simulink model "afe_abc_inv_psm"  (R2025b)
settings: Solver=ode1  StartTime=0.0  StopTime=simlength  FixedStep=tc  MaxStep=tc
values from neighbouring files (symbols this model uses):
  Adrso = eye(2) + Arso*ts_afe    [init_model.m]
  afe_pwm_phase_shift_mod1 = 0    [init_model.m]
  afe_pwm_phase_shift_mod2 = 0    [init_model.m]
  Aresd = eye(2) + Ares*ts_afe    [init_model.m]
  Bresd = Bres*ts_afe    [init_model.m]
  Cresd = Cres    [init_model.m]
  Crso = [1 0]    [init_model.m]
  CTRPIFF_CLIP_RELEASE = 0.001    [init_model.m]
  deepNEGeta = 0.5    [init_model.m]
  deepNEGxi = 0    [init_model.m]
  deepPOSxi = 0.5    [init_model.m]
  emf_fb_p = 0.2    [init_model.m]
  emf_fb_p_ccaller_1 = emf_fb_p    (= 0.2)    [init_model.m]
  emf_fb_p_ccaller_2 = emf_fb_p    (= 0.2)    [init_model.m]
  emf_p = emf_fb_p*4/10    (= 0.08)    [init_model.m]
  emf_p_ccaller_1 = emf_fb_p_ccaller_1*4/10    (= 0.08)    [init_model.m]
  emf_p_ccaller_2 = emf_fb_p_ccaller_2*4/10    (= 0.08)    [init_model.m]
  g0_161Hz = fcut_161Hz_flt * ts_afe * 2*pi    (= 0.126449104307)    [init_model.m]
  g0_1Hz = fcut_1Hz_flt * ts_afe * 2*pi    (= 0.000785398163397)    [init_model.m]
  g0_500Hz = fcut_500Hz_flt * ts_afe * 2*pi    (= 0.392699081699)    [init_model.m]
  g1_161Hz = 1 - g0_161Hz    (= 0.873550895693)    [init_model.m]
  g1_1Hz = 1 - g0_1Hz    (= 0.999214601837)    [init_model.m]
  g1_500Hz = 1 - g0_500Hz    (= 0.607300918301)    [init_model.m]
  i_grid_neg_eta_lim = 0.5    [init_model.m]
  i_grid_neg_eta_red_lim = 0.1    [init_model.m]
  i_grid_neg_xi_lim = 0.5    [init_model.m]
  i_grid_neg_xi_red_lim = 0.1    [init_model.m]
  i_grid_pos_eta_lim = 1    [init_model.m]
  i_grid_pos_eta_red_lim = 0.1    [init_model.m]
  id_lim = 0.35    [init_model.m]
  ieta_neg_ref_lim = 0.5    [init_model.m]
  ieta_pos_ref_lim = 1.0    (= 1)    [init_model.m]
  Igrid_phase_normalization_factor = 250e3/Vphase2/3/0.9*sqrt(2)    [init_model.m]
  inv_pwm_phase_shift_mod1 = 0    [init_model.m]
  iq_lim = 1.4    [init_model.m]
  ixi_pos_ref_lim = 1.6    [init_model.m]
  k_frt_ref = 2    [init_model.m]
  kg = Kobs(1)    [init_model.m]
  ki_afe = 45    [init_model.m]
  ki_align = 0.1    [init_model.m]
  ki_i = 18    [init_model.m]
  ki_rc_neg_grid = ki_rc_grid    (= 35)    [init_model.m]
  ki_rc_pos_grid = ki_rc_grid    (= 35)    [init_model.m]
  ki_vs = 35    [init_model.m]
  ki_w = 18    [init_model.m]
  kp_afe = 0.6    [init_model.m]
  kp_align = 0.6    [init_model.m]
  kp_i = 0.25    [init_model.m]
  kp_rc_neg_grid = kp_rc_grid    (= 0.35)    [init_model.m]
  kp_rc_pos_grid = kp_rc_grid    (= 0.35)    [init_model.m]
  kp_vs = 0.85    [init_model.m]
  kp_w = 2.5    [init_model.m]
  kw = Kobs(2)    [init_model.m]
  l1 = Kd(2)    [init_model.m]
  l2 = Kd(1)    [init_model.m]
  Ldrso = acker(Adrso',Crso',polesdrso)'    [init_model.m]
  lim_down_align = -0.2    [init_model.m]
  lim_up_align = 0.2    [init_model.m]
  mavarage_filter_frequency_base_order = 2    [init_model.m]
  motorc_m_scale = 2/3*Vdc_bez/ubez    [init_model.m]
  n1 = rms_perios/f_grid/ts_afe    [init_model.m]
  n10 = rms_perios/f_grid/ts_afe    [init_model.m]
  number_of_modules = 2    [init_model.m]
  omega_m_sim = omega_m_bez    [init_model.m]
  pll_i1 = 80    [init_model.m]
  pll_i1_ddsrt = pll_i1/2    (= 40)    [init_model.m]
  pll_p = 1    [init_model.m]
  pll_p_ddsrt = pll_p/2    (= 0.5)    [init_model.m]
  pll_p_frt = 0.2    [init_model.m]
  settle_time = 0.15    [init_model.m]
  simlength = 2    [init_model.m]
  start_time_LVRT = 2.0    (= 2)    [init_model.m]
  tc = ts_afe/200    (= 6.25e-07)    [init_model.m]
  time_aux_power_supply_fault = 1e3    (= 1000)    [init_model.m]
  time_gain_afe_module_1 = 1.0    (= 1)    [init_model.m]
  time_gain_afe_module_2 = 1.0    (= 1)    [init_model.m]
  time_gain_inv_module_1 = 1.0    (= 1)    [init_model.m]
  time_gain_inv_module_2 = 1.0    (= 1)    [init_model.m]
  time_phase_fault = 1e3    (= 1000)    [init_model.m]
  time_start_motor_control = 0.035    [init_model.m]
  transmission_delay = 125e-6*2    (= 0.00025)    [init_model.m]
  ts_afe = 1/fPWM_AFE/2    (= 0.000125)    [init_model.m]
  ts_inv = 1/fPWM_INV/2    (= 0.000125)    [init_model.m]
  Vdc_norm_ref = Vdc_ref/Vdc_nom    [init_model.m]
  Vdc_ref = 1070    [init_model.m]
  Vgrid_phase_normalization_factor = Vphase2*sqrt(2)    [init_model.m]
  w_grid = 2*pi*f_grid    [init_model.m]
undefined symbols (not defined in the file or in its folder): Amplitude_U, Amplitude_V, Amplitude_W, end_time_LVRT, ibez, La, Lb, Ld_norm, Lq_norm, Ls_norm, magnitude, omega_bez, omega_grid_emulator_nom, omega_grid_nom, omega_m_bez, Phase_shift, psi_bez, psi_m, psi_m_norm, rpm_base, rpm_bez, Rs, Rs_norm, t_ramp, tau_bez, torque_base, ubez, ugrid_factor, V_phase_normalization_factor, Vdc_bez, Vemu_ref_norm, vn_eta_pu, vn_xi_pu, vp_xi_pu
libraries: fl_lib x215, nesl_utility x107, simulink x22, cstblocks x20, threephase_inductor_lib x4, three_phase_pwm_modulator x4, single_phase_transformer_lib x3, power_meter_iec x1, flexshaft_lib x1, psm x1
(part 5 of 18)

== system afe_abc_inv_psm/afe_abc_inv_psm_mod2/inverter/inverter ==
  duties_uvw : Inport
  Bus Selector : BusSelector  OutputSignals=gate_cmd_Q1,gate_cmd_Q2,gate_cmd_Q3,gate_cmd_Q4,gate_cmd_Q5,gate_cmd_Q6
  Current Sensor1 : fl_lib/Electrical/Electrical Sensors/Current Sensor
  Product{,1..5} (6 alike) : Product
  Simulink-PS Converter{,1..5} (6 alike) : nesl_utility/Simulink-PS Converter  PhysicalDomain=network_engine_domain  SubClassName=ps_input  LeftPortType=input  RightPortType=output  PseudoPeriodic=off  Frequencies=[]  NoiseDistribution=none  NoiseParameters=[]  Unit=1  AffineConversion=on  FilteringAndDerivatives=provide  SimscapeFilterOrder=1  InputFilterTimeConstant=0.001  UdotUserProvided=0
  Step : Step  Time=time_aux_power_supply_fault  Before=1  After=0  SampleTime=0
  ileg_dc_inv : nesl_utility/PS-Simulink Converter  PhysicalDomain=network_engine_domain  SubClassName=ps_output  LeftPortType=input  RightPortType=output  PseudoPeriodic=off  Frequencies=[]  VectorFormat=1-D array  Unit=A  AffineConversion=on
  sv_pwm : Subsystem
  switch_1 : Subsystem
      settings: PortSchema="{\"entries\":[{\"content\":{\"sides\":[{\"content\":{\"connectorIds\":[\"LConn1\"]},\"type\":\"ConnectorPlacement.EquallySpacedRectSide\",\"uuid\":\"9277da8d-d460-43e6-8478-dd662f15d226\"},{\"content\":{\"connectorIds\":[],\"side\":\"RIGHT\"},\"type\":\"ConnectorPlacement.EquallySpacedRectSide\",\"uuid\":\"a7ece396-f1d9-4f4f-a05b-db1fc65d6e1d\"},{\"content\":{\"connectorIds\":[\"LConn2\"],\"side\":\"TOP\"},\"type\":\"ConnectorPlacement.EquallySpacedRectSide\",\"uuid\":\"fdd70777-e9cf-4317-afb6-cae87f75d5b0\"},{\"content\":{\"connectorIds\":[\"RConn1\"],\"side\":\"BOTTOM\"},\"type\":\"ConnectorPlacement.EquallySpacedRectSide\",\"uuid\":\"2353ed68-b1a1-4775-9ca9-31e268d5443b\"}]},\"type\":\"ConnectorPlacement.EquallySpacedConnector\",\"uuid\":\"d5479f4c-4e65-4791-adcb-73df11f88590\"}],\"packageUris\":[\"http://schema.mathworks.com/mf0/Connector/R2020b\"],\"version\":\"1.0\"}"
  switch_2 : Subsystem
      settings: PortSchema="{\"entries\":[{\"content\":{\"sides\":[{\"content\":{\"connectorIds\":[\"LConn1\"]},\"type\":\"ConnectorPlacement.EquallySpacedRectSide\",\"uuid\":\"9277da8d-d460-43e6-8478-dd662f15d226\"},{\"content\":{\"connectorIds\":[],\"side\":\"RIGHT\"},\"type\":\"ConnectorPlacement.EquallySpacedRectSide\",\"uuid\":\"a7ece396-f1d9-4f4f-a05b-db1fc65d6e1d\"},{\"content\":{\"connectorIds\":[\"LConn2\"],\"side\":\"TOP\"},\"type\":\"ConnectorPlacement.EquallySpacedRectSide\",\"uuid\":\"fdd70777-e9cf-4317-afb6-cae87f75d5b0\"},{\"content\":{\"connectorIds\":[\"RConn1\"],\"side\":\"BOTTOM\"},\"type\":\"ConnectorPlacement.EquallySpacedRectSide\",\"uuid\":\"2353ed68-b1a1-4775-9ca9-31e268d5443b\"}]},\"type\":\"ConnectorPlacement.EquallySpacedConnector\",\"uuid\":\"d5479f4c-4e65-4791-adcb-73df11f88590\"}],\"packageUris\":[\"http://schema.mathworks.com/mf0/Connector/R2020b\"],\"version\":\"1.0\"}"
  switch_3 : Subsystem
      settings: PortSchema="{\"entries\":[{\"content\":{\"sides\":[{\"content\":{\"connectorIds\":[\"LConn1\"]},\"type\":\"ConnectorPlacement.EquallySpacedRectSide\",\"uuid\":\"9277da8d-d460-43e6-8478-dd662f15d226\"},{\"content\":{\"connectorIds\":[],\"side\":\"RIGHT\"},\"type\":\"ConnectorPlacement.EquallySpacedRectSide\",\"uuid\":\"a7ece396-f1d9-4f4f-a05b-db1fc65d6e1d\"},{\"content\":{\"connectorIds\":[\"LConn2\"],\"side\":\"TOP\"},\"type\":\"ConnectorPlacement.EquallySpacedRectSide\",\"uuid\":\"fdd70777-e9cf-4317-afb6-cae87f75d5b0\"},{\"content\":{\"connectorIds\":[\"RConn1\"],\"side\":\"BOTTOM\"},\"type\":\"ConnectorPlacement.EquallySpacedRectSide\",\"uuid\":\"2353ed68-b1a1-4775-9ca9-31e268d5443b\"}]},\"type\":\"ConnectorPlacement.EquallySpacedConnector\",\"uuid\":\"d5479f4c-4e65-4791-adcb-73df11f88590\"}],\"packageUris\":[\"http://schema.mathworks.com/mf0/Connector/R2020b\"],\"version\":\"1.0\"}"
  switch_4 : Subsystem
      settings: PortSchema="{\"entries\":[{\"content\":{\"sides\":[{\"content\":{\"connectorIds\":[\"LConn1\"]},\"type\":\"ConnectorPlacement.EquallySpacedRectSide\",\"uuid\":\"9277da8d-d460-43e6-8478-dd662f15d226\"},{\"content\":{\"connectorIds\":[],\"side\":\"RIGHT\"},\"type\":\"ConnectorPlacement.EquallySpacedRectSide\",\"uuid\":\"a7ece396-f1d9-4f4f-a05b-db1fc65d6e1d\"},{\"content\":{\"connectorIds\":[\"LConn2\"],\"side\":\"TOP\"},\"type\":\"ConnectorPlacement.EquallySpacedRectSide\",\"uuid\":\"fdd70777-e9cf-4317-afb6-cae87f75d5b0\"},{\"content\":{\"connectorIds\":[\"RConn1\"],\"side\":\"BOTTOM\"},\"type\":\"ConnectorPlacement.EquallySpacedRectSide\",\"uuid\":\"2353ed68-b1a1-4775-9ca9-31e268d5443b\"}]},\"type\":\"ConnectorPlacement.EquallySpacedConnector\",\"uuid\":\"d5479f4c-4e65-4791-adcb-73df11f88590\"}],\"packageUris\":[\"http://schema.mathworks.com/mf0/Connector/R2020b\"],\"version\":\"1.0\"}"
  switch_5 : Subsystem
      settings: PortSchema="{\"entries\":[{\"content\":{\"sides\":[{\"content\":{\"connectorIds\":[\"LConn1\"]},\"type\":\"ConnectorPlacement.EquallySpacedRectSide\",\"uuid\":\"9277da8d-d460-43e6-8478-dd662f15d226\"},{\"content\":{\"connectorIds\":[],\"side\":\"RIGHT\"},\"type\":\"ConnectorPlacement.EquallySpacedRectSide\",\"uuid\":\"a7ece396-f1d9-4f4f-a05b-db1fc65d6e1d\"},{\"content\":{\"connectorIds\":[\"LConn2\"],\"side\":\"TOP\"},\"type\":\"ConnectorPlacement.EquallySpacedRectSide\",\"uuid\":\"fdd70777-e9cf-4317-afb6-cae87f75d5b0\"},{\"content\":{\"connectorIds\":[\"RConn1\"],\"side\":\"BOTTOM\"},\"type\":\"ConnectorPlacement.EquallySpacedRectSide\",\"uuid\":\"2353ed68-b1a1-4775-9ca9-31e268d5443b\"}]},\"type\":\"ConnectorPlacement.EquallySpacedConnector\",\"uuid\":\"d5479f4c-4e65-4791-adcb-73df11f88590\"}],\"packageUris\":[\"http://schema.mathworks.com/mf0/Connector/R2020b\"],\"version\":\"1.0\"}"
  switch_6 : Subsystem
      settings: PortSchema="{\"entries\":[{\"content\":{\"sides\":[{\"content\":{\"connectorIds\":[\"LConn1\"]},\"type\":\"ConnectorPlacement.EquallySpacedRectSide\",\"uuid\":\"9277da8d-d460-43e6-8478-dd662f15d226\"},{\"content\":{\"connectorIds\":[],\"side\":\"RIGHT\"},\"type\":\"ConnectorPlacement.EquallySpacedRectSide\",\"uuid\":\"a7ece396-f1d9-4f4f-a05b-db1fc65d6e1d\"},{\"content\":{\"connectorIds\":[\"LConn2\"],\"side\":\"TOP\"},\"type\":\"ConnectorPlacement.EquallySpacedRectSide\",\"uuid\":\"fdd70777-e9cf-4317-afb6-cae87f75d5b0\"},{\"content\":{\"connectorIds\":[\"RConn1\"],\"side\":\"BOTTOM\"},\"type\":\"ConnectorPlacement.EquallySpacedRectSide\",\"uuid\":\"2353ed68-b1a1-4775-9ca9-31e268d5443b\"}]},\"type\":\"ConnectorPlacement.EquallySpacedConnector\",\"uuid\":\"d5479f4c-4e65-4791-adcb-73df11f88590\"}],\"packageUris\":[\"http://schema.mathworks.com/mf0/Connector/R2020b\"],\"version\":\"1.0\"}"
  u : PMIOPort  Side=Left
  v : PMIOPort  Port=2  Side=Left
  w : PMIOPort  Port=3  Side=Left
  V+ : PMIOPort  Port=4  Side=Right
  V- : PMIOPort  Port=5  Side=Right
  tag scope: ileg_dc_inv_mod2=global
  wires:
  duties_uvw/1 -> sv_pwm/1(duties_uvw)
  Bus Selector/6 -> Product5/2  "<gate_cmd_Q6>"
  Bus Selector/5 -> Product4/2  "<gate_cmd_Q5>"
  Bus Selector/4 -> Product3/2  "<gate_cmd_Q4>"
  Bus Selector/3 -> Product2/2  "<gate_cmd_Q3>"
  Bus Selector/2 -> Product1/2  "<gate_cmd_Q2>"
  Bus Selector/1 -> Product/2  "<gate_cmd_Q1>"
  Step/1 -> Product1/1, Product/1, Product2/1, Product3/1, Product4/1, Product5/1
  Product1/1 -> [I2]
  Product2/1 -> [I3]
  Product5/1 -> [I6]
  Product4/1 -> [I5]
  Product3/1 -> [I4]
  Product/1 -> [I1]
  ileg_dc_inv/1 -> [ileg_dc_inv_mod2]
  sv_pwm/1(gate_cmds) -> Bus Selector/1
  [I6] -> Simulink-PS Converter5/1
  [I5] -> Simulink-PS Converter4/1
  [I4] -> Simulink-PS Converter3/1
  [I3] -> Simulink-PS Converter2/1
  [I2] -> Simulink-PS Converter1/1
  [I1] -> Simulink-PS Converter/1
  connections:
  Current Sensor1/RConn1 -- ileg_dc_inv/LConn1
  switch_1/LConn2 -- Current Sensor1/RConn2
  switch_5/RConn1 -- switch_6/LConn2 -- w/RConn1
  switch_3/RConn1 -- switch_4/LConn2 -- v/RConn1
  switch_1/RConn1 -- switch_2/LConn2 -- u/RConn1
  switch_6/LConn1 -- Simulink-PS Converter5/RConn1
  switch_5/LConn1 -- Simulink-PS Converter4/RConn1
  switch_4/LConn1 -- Simulink-PS Converter3/RConn1
  switch_3/LConn1 -- Simulink-PS Converter2/RConn1
  switch_2/LConn1 -- Simulink-PS Converter1/RConn1
  switch_1/LConn1 -- Simulink-PS Converter/RConn1
  switch_4/RConn1 -- switch_6/RConn1 -- switch_2/RConn1 -- V-/RConn1
  switch_3/LConn2 -- switch_5/LConn2 -- V+/RConn1 -- Current Sensor1/LConn1

== system afe_abc_inv_psm/grid/grid_emulator/3ph_Dyg ==
  Electrical Reference1 : fl_lib/Electrical/Electrical Elements/Electrical Reference
  ph1 : single_phase_transformer_lib/single phase transformer  Lm=Lmu2_trafo H  n1=50*sqrt(3)  n2=50  Rd1=0 Ohm  Rd2=Rd2_trafo Ohm  Ld1=0 H  Ld2=Ld2_trafo H  Rfe=Rm2_trafo Ohm  phi_specify=off  phi_priority=None  phi=0 V*s  phi_nominal_specify=off  phi_nominal_value=1  phi_nominal_unit=V*s  i1_specify=off  i1_priority=None  i1=0 A  i1_nominal_specify=off  i1_nominal_value=1  i1_nominal_unit=A  i2_specify=off  i2_priority=None  i2=0 A  i2_nominal_specify=off  i2_nominal_value=1  i2_nominal_unit=A  ife_specify=off  ife_priority=None  ife=0 A  ife_nominal_specify=off  ife_nominal_value=1  ife_nominal_unit=A  u1_specify=off  u1_priority=None  u1=0 V  u1_nominal_specify=off  u1_nominal_value=1  u1_nominal_unit=V  u2_specify=off  u2_priority=None  u2=0 V  u2_nominal_specify=off  u2_nominal_value=1  u2_nominal_unit=V
      settings: InternalSimscapePortConfiguration="{\"Bottom\":[],\"Left\":[{\"id\":\"u1_p\",\"label\":\"u1(+)\",\"type\":\"foundation.electrical.electrical\"},{\"id\":\"u1_n\",\"label\":\"u1(-)\",\"type\":\"foundation.electrical.electrical\"}],\"Right\":[{\"id\":\"u2_p\",\"label\":\"u2(+)\",\"type\":\"foundation.electrical.electrical\"},{\"id\":\"u2_n\",\"label\":\"u2(-)\",\"type\":\"foundation.electrical.electrical\"}],\"Top\":[]}"
  ph2 : single_phase_transformer_lib/single phase transformer  Lm=Lmu2_trafo H  n1=50*sqrt(3)  n2=50  Rd1=0 Ohm  Rd2=Rd2_trafo Ohm  Ld1=0 H  Ld2=Ld2_trafo H  Rfe=Rm2_trafo Ohm  phi_specify=off  phi_priority=None  phi=0 V*s  phi_nominal_specify=off  phi_nominal_value=1  phi_nominal_unit=V*s  i1_specify=off  i1_priority=None  i1=0 A  i1_nominal_specify=off  i1_nominal_value=1  i1_nominal_unit=A  i2_specify=off  i2_priority=None  i2=0 A  i2_nominal_specify=off  i2_nominal_value=1  i2_nominal_unit=A  ife_specify=off  ife_priority=None  ife=0 A  ife_nominal_specify=off  ife_nominal_value=1  ife_nominal_unit=A  u1_specify=off  u1_priority=None  u1=0 V  u1_nominal_specify=off  u1_nominal_value=1  u1_nominal_unit=V  u2_specify=off  u2_priority=None  u2=0 V  u2_nominal_specify=off  u2_nominal_value=1  u2_nominal_unit=V
      settings: InternalSimscapePortConfiguration="{\"Bottom\":[],\"Left\":[{\"id\":\"u1_p\",\"label\":\"u1(+)\",\"type\":\"foundation.electrical.electrical\"},{\"id\":\"u1_n\",\"label\":\"u1(-)\",\"type\":\"foundation.electrical.electrical\"}],\"Right\":[{\"id\":\"u2_p\",\"label\":\"u2(+)\",\"type\":\"foundation.electrical.electrical\"},{\"id\":\"u2_n\",\"label\":\"u2(-)\",\"type\":\"foundation.electrical.electrical\"}],\"Top\":[]}"
  ph3 : single_phase_transformer_lib/single phase transformer  Lm=Lmu2_trafo H  n1=50*sqrt(3)  n2=50  Rd1=0 Ohm  Rd2=Rd2_trafo Ohm  Ld1=0 H  Ld2=Ld2_trafo H  Rfe=Rm2_trafo Ohm  phi_specify=off  phi_priority=None  phi=0 V*s  phi_nominal_specify=off  phi_nominal_value=1  phi_nominal_unit=V*s  i1_specify=off  i1_priority=None  i1=0 A  i1_nominal_specify=off  i1_nominal_value=1  i1_nominal_unit=A  i2_specify=off  i2_priority=None  i2=0 A  i2_nominal_specify=off  i2_nominal_value=1  i2_nominal_unit=A  ife_specify=off  ife_priority=None  ife=0 A  ife_nominal_specify=off  ife_nominal_value=1  ife_nominal_unit=A  u1_specify=off  u1_priority=None  u1=0 V  u1_nominal_specify=off  u1_nominal_value=1  u1_nominal_unit=V  u2_specify=off  u2_priority=None  u2=0 V  u2_nominal_specify=off  u2_nominal_value=1  u2_nominal_unit=V
      settings: InternalSimscapePortConfiguration="{\"Bottom\":[],\"Left\":[{\"id\":\"u1_p\",\"label\":\"u1(+)\",\"type\":\"foundation.electrical.electrical\"},{\"id\":\"u1_n\",\"label\":\"u1(-)\",\"type\":\"foundation.electrical.electrical\"}],\"Right\":[{\"id\":\"u2_p\",\"label\":\"u2(+)\",\"type\":\"foundation.electrical.electrical\"},{\"id\":\"u2_n\",\"label\":\"u2(-)\",\"type\":\"foundation.electrical.electrical\"}],\"Top\":[]}"
  ua : PMIOPort  Side=Right
  ub : PMIOPort  Port=2  Side=Right
  uc : PMIOPort  Port=3  Side=Right
  Ua : PMIOPort  Port=4  Side=Left
  Ub : PMIOPort  Port=5  Side=Left
  Uc : PMIOPort  Port=6  Side=Left
  connections:
  Electrical Reference1/LConn1 -- ph3/RConn2 -- ph2/RConn2 -- ph1/RConn2
  ph3/RConn1 -- uc/RConn1
  ph1/LConn1 -- ph3/LConn2 -- Ua/RConn1
  ph1/RConn1 -- ua/RConn1
  ph2/RConn1 -- ub/RConn1
  ph1/LConn2 -- ph2/LConn1 -- Ub/RConn1
  Uc/RConn1 -- ph3/LConn1 -- ph2/LConn2

== system afe_abc_inv_psm/grid/grid_emulator/grid_emulator ==
  phase_gen : Subsystem
  voltage_reference : Subsystem
  voltage_source : Subsystem
  Vma : Outport
  Vmb : Outport  Port=2
  Vmc : Outport  Port=3
  wires:
  phase_gen/1(grid_emu_phase) -> voltage_reference/1(grid_emu_phase)  "grid_emu_phase"
  voltage_source/2(vn_xi) -> voltage_reference/3(Vxi_n)
  voltage_source/1(vp_xi) -> voltage_reference/2(Vxi_p)
  voltage_source/3(vn_eta) -> voltage_reference/4(Veta_n)
  voltage_reference/3(V3_ref) -> Vmc/1
  voltage_reference/1(V1_ref) -> Vma/1
  voltage_reference/2(V2_ref) -> Vmb/1

== system afe_abc_inv_psm/grid/grid_emulator/threephase_vi_measures ==
  Bus Creator : BusCreator  Inputs=6
  Current Sensor : fl_lib/Electrical/Electrical Sensors/Current Sensor
  Current Sensor1 : fl_lib/Electrical/Electrical Sensors/Current Sensor
  Current Sensor2 : fl_lib/Electrical/Electrical Sensors/Current Sensor
  Electrical Reference1 : fl_lib/Electrical/Electrical Elements/Electrical Reference
  Voltage Sensor : fl_lib/Electrical/Electrical Sensors/Voltage Sensor
  Voltage Sensor1 : fl_lib/Electrical/Electrical Sensors/Voltage Sensor
  Voltage Sensor2 : fl_lib/Electrical/Electrical Sensors/Voltage Sensor
  i : Selector  InputPortWidth=6  IndexOptions=Index vector (dialog)  Indices=[4 5 6]  OutputSizes=1
  i_line_abc/u_line_abc : Scope  NumInputPorts=2
      settings: SampleTime=tc  ActiveDisplayYMinimum=-772.33923102813571  ActiveDisplayYMaximum=762.04131991148563  DataLoggingVariableName=ScopeData2
  ia_grid : nesl_utility/PS-Simulink Converter  PhysicalDomain=network_engine_domain  SubClassName=ps_output  LeftPortType=input  RightPortType=output  PseudoPeriodic=off  Frequencies=[]  VectorFormat=1-D array  Unit=A  AffineConversion=off
  ib_grid : nesl_utility/PS-Simulink Converter  PhysicalDomain=network_engine_domain  SubClassName=ps_output  LeftPortType=input  RightPortType=output  PseudoPeriodic=off  Frequencies=[]  VectorFormat=1-D array  Unit=A  AffineConversion=off
  ic_grid : nesl_utility/PS-Simulink Converter  PhysicalDomain=network_engine_domain  SubClassName=ps_output  LeftPortType=input  RightPortType=output  PseudoPeriodic=off  Frequencies=[]  VectorFormat=1-D array  Unit=A  AffineConversion=off
  u : Selector  InputPortWidth=6  IndexOptions=Index vector (dialog)  Indices=[1 2 3]  OutputSizes=1
  ua_grid : nesl_utility/PS-Simulink Converter  PhysicalDomain=network_engine_domain  SubClassName=ps_output  LeftPortType=input  RightPortType=output  PseudoPeriodic=off  Frequencies=[]  VectorFormat=1-D array  Unit=V  AffineConversion=off
  ub_grid : nesl_utility/PS-Simulink Converter  PhysicalDomain=network_engine_domain  SubClassName=ps_output  LeftPortType=input  RightPortType=output  PseudoPeriodic=off  Frequencies=[]  VectorFormat=1-D array  Unit=V  AffineConversion=off
  uc_grid : nesl_utility/PS-Simulink Converter  PhysicalDomain=network_engine_domain  SubClassName=ps_output  LeftPortType=input  RightPortType=output  PseudoPeriodic=off  Frequencies=[]  VectorFormat=1-D array  Unit=V  AffineConversion=off
  Ua : PMIOPort  Side=Left
  ua : PMIOPort  Port=2  Side=Right
  Ub : PMIOPort  Port=3  Side=Left
  ub : PMIOPort  Port=4  Side=Right
  Uc : PMIOPort  Port=5  Side=Left
  uc : PMIOPort  Port=6  Side=Right
  wires:
  Bus Creator/1 -> i/1, u/1  "vi_data"
  ib_grid/1 -> Bus Creator/5  "ib"
  ia_grid/1 -> Bus Creator/4  "ia"
  ic_grid/1 -> Bus Creator/6  "ic"
  ua_grid/1 -> Bus Creator/1  "ua"
  ub_grid/1 -> Bus Creator/2  "ub"
  uc_grid/1 -> Bus Creator/3  "uc"
  i/1 -> i_line_abc/u_line_abc/1
  u/1 -> i_line_abc/u_line_abc/2
  connections:
  Current Sensor1/LConn1 -- Ub/RConn1 -- Voltage Sensor1/LConn1
  Electrical Reference1/LConn1 -- Voltage Sensor/RConn2 -- Voltage Sensor2/RConn2 -- Voltage Sensor1/RConn2
  Voltage Sensor/RConn1 -- ua_grid/LConn1
  Current Sensor/RConn2 -- ua/RConn1
  Voltage Sensor1/RConn1 -- ub_grid/LConn1
  Voltage Sensor2/LConn1 -- Current Sensor2/LConn1 -- Uc/RConn1
  Current Sensor/LConn1 -- Ua/RConn1 -- Voltage Sensor/LConn1
  Current Sensor1/RConn2 -- ub/RConn1
  Voltage Sensor2/RConn1 -- uc_grid/LConn1
  ib_grid/LConn1 -- Current Sensor1/RConn1
  ia_grid/LConn1 -- Current Sensor/RConn1
  ic_grid/LConn1 -- Current Sensor2/RConn1
  Current Sensor2/RConn2 -- uc/RConn1

== system afe_abc_inv_psm/afe_abc_inv_psm_mod1/AFE_control/afe_control/FRT-VDE4110 ==
  FRT-Detection : Subsystem
  FRT-PosNegReactiveCurrentReferences : Subsystem
  frt_detection_output : Scope  NumInputPorts=3
      settings: ActiveDisplayYMinimum=-0.125  ActiveDisplayYMaximum=1.125
  tag scope: frt_active_mod1=global, pwr_lim_enable_mod1=global
  wires:
  [v_grid_pos_xi_avg_mod1] -> FRT-PosNegReactiveCurrentReferences/1(In1)
  [v_grid_neg_xi_avg_mod1] -> FRT-PosNegReactiveCurrentReferences/3(In3)
  [v_grid_neg_eta_avg_mod1] -> FRT-PosNegReactiveCurrentReferences/4(In4)
  [v_grid_pos_eta_avg_mod1] -> FRT-PosNegReactiveCurrentReferences/2(In2)
  FRT-Detection/4(frt_active) -> frt_detection_output/2, [frt_active_mod1]  "frt_active"
  FRT-Detection/5(pwr_lim_enable) -> frt_detection_output/3, [pwr_lim_enable_mod1]  "pwr_lim_enable"
  FRT-Detection/2(frt_state) -> frt_detection_output/1  "frt_state"

== system afe_abc_inv_psm/afe_abc_inv_psm_mod1/AFE_control/afe_control/current_ctrl ==
  i_xi_ref : Inport
  is_abc_pu : Inport  Port=2
  Demux : Demux  Outputs=3
  Inner Loop Current Control : Subsystem
  current_transformation : Subsystem
  xieta2abc : Subsystem
  uab_out : Outport
  wires:
  Demux/1 -> current_transformation/1(is_a_pu)  "is_a"
  Demux/2 -> current_transformation/2(is_b_pu)  "is_b"
  Demux/3 -> current_transformation/3(is_c_pu)  "is_c"
  is_abc_pu/1 -> Demux/1
  [gamma_grid_pll_mod1] -> xieta2abc/5(gamma)
  xieta2abc/1(i_abc) -> Inner Loop Current Control/1(In1)
  [isd_abc_pu_mod1] -> Inner Loop Current Control/2(is_abc)
  Inner Loop Current Control/1(uab) -> uab_out/1
  i_xi_ref/1 -> xieta2abc/1(pos_xi)  "i_xi_ref"
  [i_stack_neg_eta_ref_mod1] -> xieta2abc/4(neg_eta)
  [i_stack_neg_xi_ref_mod1] -> xieta2abc/3(neg_xi)
  [i_stack_pos_eta_ref_mod1] -> xieta2abc/2(pos_eta)

== system afe_abc_inv_psm/afe_abc_inv_psm_mod1/AFE_control/afe_control/data_to_worspace_module_1 ==
  Bus Selector : BusSelector  OutputSignals=i_grid_pos_eta_ref,i_grid_neg_eta_ref,i_grid_neg_xi_ref
  To Workspace1 : ToWorkspace  VariableName=i_grid_pos_eta_ref_sim_mod1  SampleTime=-1
      settings: MaxDataPoints=Ns_afe
  To Workspace11 : ToWorkspace  VariableName=i_grid_pos_xi_sim_mod1  SampleTime=-1
      settings: MaxDataPoints=Ns_afe
  To Workspace13 : ToWorkspace  VariableName=i_grid_pos_eta_sim_mod1  SampleTime=-1
      settings: MaxDataPoints=Ns_afe
  To Workspace14 : ToWorkspace  VariableName=i_grid_neg_xi_sim_mod1  SampleTime=-1
      settings: MaxDataPoints=Ns_afe
  To Workspace15 : ToWorkspace  VariableName=i_grid_neg_eta_sim_mod1  SampleTime=-1
      settings: MaxDataPoints=Ns_afe
  To Workspace16 : ToWorkspace  VariableName=u_grid_pos_xi_sim_mod1  SampleTime=-1
      settings: MaxDataPoints=Ns_afe
  To Workspace17 : ToWorkspace  VariableName=u_grid_pos_eta_sim_mod1  SampleTime=-1
      settings: MaxDataPoints=Ns_afe
  To Workspace18 : ToWorkspace  VariableName=u_grid_neg_xi_sim_mod1  SampleTime=-1
      settings: MaxDataPoints=Ns_afe
  To Workspace19 : ToWorkspace  VariableName=u_grid_neg_eta_sim_mod1  SampleTime=-1
      settings: MaxDataPoints=Ns_afe
  To Workspace2 : ToWorkspace  VariableName=i_grid_neg_xi_ref_sim_mod1  SampleTime=-1
      settings: MaxDataPoints=Ns_afe
  To Workspace3 : ToWorkspace  VariableName=i_grid_neg_eta_ref_sim_mod1  SampleTime=-1
      settings: MaxDataPoints=Ns_afe
  wires:
  [i_grid_pos_eta_avg_mod1] -> To Workspace13/1
  [i_grid_pos_xi_avg_mod1] -> To Workspace11/1
  [i_grid_neg_xi_avg_mod1] -> To Workspace14/1
  [i_grid_neg_eta_avg_mod1] -> To Workspace15/1
  [v_grid_pos_xi_avg_mod1] -> To Workspace16/1
  [v_grid_neg_eta_avg_mod1] -> To Workspace19/1
  [v_grid_pos_eta_avg_mod1] -> To Workspace17/1
  [v_grid_neg_xi_avg_mod1] -> To Workspace18/1
  [i_grid_seq_ref_mod1] -> Bus Selector/1
  Bus Selector/1 -> To Workspace1/1  "<i_grid_pos_eta_ref>"
  Bus Selector/2 -> To Workspace3/1  "<i_grid_neg_eta_ref>"
  Bus Selector/3 -> To Workspace2/1  "<i_grid_neg_xi_ref>"

== system afe_abc_inv_psm/afe_abc_inv_psm_mod1/AFE_control/afe_control/grid_current_sequences_and_reactive_pwr_ctrl ==
  ig_abc_pu : Inport
  current_sequence_avg : Subsystem
  grid_current_sampling_and_alpha_beta_transformation : Subsystem
  i_alphabeta2xieta : Subsystem
  sequences_current_control : Subsystem
  tag scope: i_grid_neg_eta_avg_mod1=global, i_grid_neg_xi_avg_mod1=global, i_grid_pos_eta_avg_mod1=global, i_grid_pos_xi_avg_mod1=global
  wires:
  i_alphabeta2xieta/1(xi) -> current_sequence_avg/1(i_grid_pos_xi)
  i_alphabeta2xieta/3(v_grid_neg_xi) -> current_sequence_avg/3(i_grid_neg_xi)
  i_alphabeta2xieta/4(e) -> current_sequence_avg/4(i_grid_neg_eta)
  current_sequence_avg/4(i_grid_neg_eta_avg) -> sequences_current_control/4(i_neg_eta), [i_grid_neg_eta_avg_mod1]
  ig_abc_pu/1 -> grid_current_sampling_and_alpha_beta_transformation/1(ig_abc)
  i_alphabeta2xieta/2(v_grid_pos_eta) -> current_sequence_avg/2(i_grid_pos_eta)
  current_sequence_avg/1(i_grid_pos_xi_avg) -> [i_grid_pos_xi_avg_mod1], sequences_current_control/1(i_pos_xi)
  current_sequence_avg/2(i_grid_pos_eta_avg) -> [i_grid_pos_eta_avg_mod1], sequences_current_control/2(i_pos_eta)
  [gamma_grid_pll_mod1] -> i_alphabeta2xieta/3(gamma)
  grid_current_sampling_and_alpha_beta_transformation/2(i_grid_beta) -> i_alphabeta2xieta/2(beta)
  grid_current_sampling_and_alpha_beta_transformation/1(i_grid_alpha) -> i_alphabeta2xieta/1(alpha)
  current_sequence_avg/3(i_grid_neg_xi_avg) -> sequences_current_control/3(i_neg_xi), [i_grid_neg_xi_avg_mod1]

== system afe_abc_inv_psm/afe_abc_inv_psm_mod1/AFE_control/afe_control/grid_voltage_phase_lock_loops ==
  ug_abc_pu : Inport
  DDSRF-PLL : Subsystem  Commented=on
  To Workspace1 : ToWorkspace  VariableName=gamma_grid_ddsrf_pll_sim_mod1  SampleTime=-1
      settings: MaxDataPoints=Ns_afe
  To Workspace2 : ToWorkspace  VariableName=omega_grid_ddsrf_pll_sim_mod1  SampleTime=-1
      settings: MaxDataPoints=Ns_afe
  To Workspace3 : ToWorkspace  VariableName=gamma_grid_dqpll_sim_mod1  SampleTime=-1
      settings: MaxDataPoints=Ns_afe
  To Workspace4 : ToWorkspace  VariableName=omega_grid_dqpll_sim_mod1  SampleTime=-1
      settings: MaxDataPoints=Ns_afe
  To Workspace5 : ToWorkspace  VariableName=gamma_grid_dqpll_ccaller_sim_mod1  SampleTime=-1
      settings: MaxDataPoints=Ns_afe
  To Workspace6 : ToWorkspace  VariableName=omega_grid_dqpll_ccaller_sim_mod1  SampleTime=-1
      settings: MaxDataPoints=Ns_afe
  Variant Source1 : VariantSource  VariantControls={use_advanced_pll == 1, use_dq_pll_ccaller_mod1 == 0, use_dq_pll_ccaller_mod1 == 1}
  Variant Source2 : VariantSource  VariantControls={use_advanced_pll == 1, use_dq_pll_ccaller_mod1 == 0, use_dq_pll_ccaller_mod1 == 1}
  dq_pll : Subsystem
  dq_pll_ccaller : Subsystem
  dqpll_ccaler : Scope  NumInputPorts=3
      settings: ActiveDisplayYMinimum=-0.88802937790751446  ActiveDisplayYMaximum=4.5431143753230572  DataLoggingVariableName=ScopeData4
  grid_plls_performance : Scope  NumInputPorts=3
      settings: ActiveDisplayYMinimum=-3.9100335923701763  ActiveDisplayYMaximum=3.915893289496164
  tag scope: gamma_grid_pll_mod1=global, omega_grid_pll_mod1=global
  wires:
  Variant Source1/1 -> [gamma_grid_pll_mod1]
  DDSRF-PLL/1(gamma_grid_ddsrf_pll) -> [gamma_grid_ddsrf_pll]
  DDSRF-PLL/2(omega_grid_ddsrf_pll) -> [omega_grid_ddsrf_pll]
  dq_pll/2(omega_grid_pu_dqpll) -> [omega_grid_pu_dqpll]
  dq_pll/1(gamma_grid_dqpll) -> [gamma_grid_dqpll]
  dq_pll_ccaller/1(gamma_hat) -> [gamma_grid_dqpll_ccaller]
  dq_pll_ccaller/2(omega_pu_hat) -> [omega_grid_dqpll_ccaller]
  [gamma_grid_ddsrf_pll] -> Variant Source1/1
  [gamma_grid_dqpll] -> Variant Source1/2
  [gamma_grid_dqpll_ccaller] -> Variant Source1/3
  [omega_grid_ddsrf_pll] -> Variant Source2/1
  [omega_grid_pu_dqpll] -> Variant Source2/2
  [omega_grid_dqpll_ccaller] -> Variant Source2/3
  Variant Source2/1 -> [omega_grid_pll_mod1]
  [gamma_grid_dqpll_ccaller] -> grid_plls_performance/3  "gamma_grid_dqpll_ccaller"
  [gamma_grid_dqpll] -> grid_plls_performance/2  "gamma_grid_dqpll"
  dq_pll_ccaller/3(dqpll_uxi) -> dqpll_ccaler/1  "uxi_n"
  dq_pll_ccaller/4(dqpll_ueta) -> dqpll_ccaler/2  "ueta_n"
  dq_pll_ccaller/5(dqpll_state) -> dqpll_ccaler/3  "dqpll_state"
  ug_abc_pu/1 -> dq_pll/1(ug_abc_pu), DDSRF-PLL/1(ug_abc_pu), dq_pll_ccaller/1(ug_abc_pu)
  [omega_grid_pll_mod1] -> grid_plls_performance/1  "omega_grid_pll_mod1"
  [gamma_grid_ddsrf_pll] -> To Workspace1/1
  [omega_grid_ddsrf_pll] -> To Workspace2/1
  [gamma_grid_dqpll] -> To Workspace3/1
  [omega_grid_pu_dqpll] -> To Workspace4/1
  [gamma_grid_dqpll_ccaller] -> To Workspace5/1
  [omega_grid_dqpll_ccaller] -> To Workspace6/1

== system afe_abc_inv_psm/afe_abc_inv_psm_mod1/AFE_control/afe_control/grid_voltage_sequences ==
  grid_voltage_sampling_and_alpha_beta_transformation : Subsystem
  v_alphabeta2xieta : Subsystem
  voltage_sequence_avg : Subsystem
  tag scope: ug_alpha_pu_mod1=global, ug_beta_pu_mod1=global, v_grid_neg_eta_avg_mod1=global, v_grid_neg_xi_avg_mod1=global, v_grid_pos_eta_avg_mod1=global, v_grid_pos_xi_avg_mod1=global
  wires:
  v_alphabeta2xieta/4(v_grid_neg_eta) -> voltage_sequence_avg/4(v_grid_neg_eta)  "neg_eta"
  v_alphabeta2xieta/2(eta) -> voltage_sequence_avg/2(v_grid_pos_eta)  "pos_eta"
  [gamma_grid_pll_mod1] -> v_alphabeta2xieta/3(gamma)
  v_alphabeta2xieta/3(v_grid_neg_xi) -> voltage_sequence_avg/3(v_grid_neg_xi)  "neg_xi"
  voltage_sequence_avg/3(v_grid_neg_xi_avg) -> [v_grid_neg_xi_avg_mod1]
  voltage_sequence_avg/2(v_grid_pos_eta_avg) -> [v_grid_pos_eta_avg_mod1]
  voltage_sequence_avg/4(v_grid_neg_eta_avg) -> [v_grid_neg_eta_avg_mod1]
  grid_voltage_sampling_and_alpha_beta_transformation/2(u_grid_beta) -> [ug_beta_pu_mod1], v_alphabeta2xieta/2(beta)
  voltage_sequence_avg/1(v_grid_pos_xi_avg) -> [v_grid_pos_xi_avg_mod1]
  v_alphabeta2xieta/1(xi) -> voltage_sequence_avg/1(v_grid_pos_xi)  "pos_xi"
  grid_voltage_sampling_and_alpha_beta_transformation/1(u_grid_alpha) -> [ug_alpha_pu_mod1], v_alphabeta2xieta/1(alpha)
  [ugd_abc_pu_mod1] -> grid_voltage_sampling_and_alpha_beta_transformation/1(v_abc)

== system afe_abc_inv_psm/afe_abc_inv_psm_mod1/AFE_control/afe_control/ig afe quantizzation and one step delay ==
  ig_abc_pu : Inport
  Demux1 : Demux  Outputs=3
  Mux1 : Mux  Inputs=3
  ig afe quantizzation and one step delay : Subsystem
  igd_abc_pu : Outport
  wires:
  Demux1/1 -> ig afe quantizzation and one step delay/1(ig_u_pu)
  Demux1/2 -> ig afe quantizzation and one step delay/2(ig_v_pu)
  ig_abc_pu/1 -> Demux1/1
  Mux1/1 -> igd_abc_pu/1
  Demux1/3 -> ig afe quantizzation and one step delay/3(ig_w_pu)
  ig afe quantizzation and one step delay/2(igd_v_pu) -> Mux1/2
  ig afe quantizzation and one step delay/1(igd_u_pu) -> Mux1/1
  ig afe quantizzation and one step delay/3(igd_w_pu) -> Mux1/3

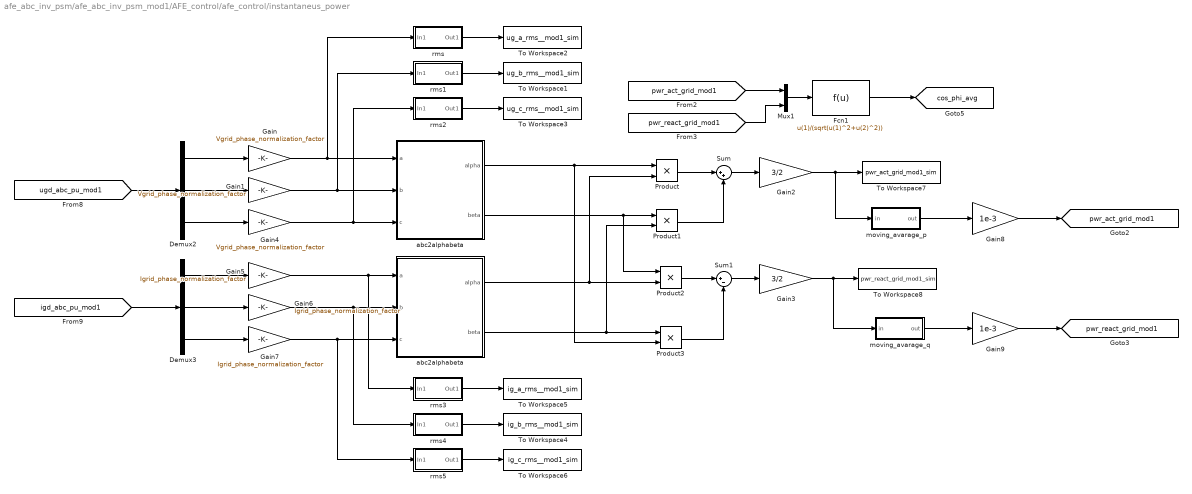
== system afe_abc_inv_psm/afe_abc_inv_psm_mod1/AFE_control/afe_control/instantaneus_power ==
  Demux2 : Demux  Outputs=3
  Demux3 : Demux  Outputs=3
  Fcn1 : Fcn  Expr=u(1)/(sqrt(u(1)^2+u(2)^2))
  Gain : Gain  Gain=Vgrid_phase_normalization_factor
  Gain1 : Gain  Gain=Vgrid_phase_normalization_factor
  Gain2 : Gain  Gain=3/2
  Gain3 : Gain  Gain=3/2
  Gain4 : Gain  Gain=Vgrid_phase_normalization_factor
  Gain5 : Gain  Gain=Igrid_phase_normalization_factor
  Gain6 : Gain  Gain=Igrid_phase_normalization_factor
  Gain7 : Gain  Gain=Igrid_phase_normalization_factor
  Gain8 : Gain  Gain=1e-3
  Gain9 : Gain  Gain=1e-3
  Mux1 : Mux  Inputs=2
  Product{,1..3} (4 alike) : Product  RndMeth=Zero
  Sum : Sum  Inputs=|++
  Sum1 : Sum  Inputs=|+-
  To Workspace1 : ToWorkspace  VariableName=ug_b_rms__mod1_sim  SampleTime=-1
      settings: MaxDataPoints=Ns_afe
  To Workspace2 : ToWorkspace  VariableName=ug_a_rms__mod1_sim  SampleTime=-1
      settings: MaxDataPoints=Ns_afe
  To Workspace3 : ToWorkspace  VariableName=ug_c_rms__mod1_sim  SampleTime=-1
      settings: MaxDataPoints=Ns_afe
  To Workspace4 : ToWorkspace  VariableName=ig_b_rms__mod1_sim  SampleTime=-1
      settings: MaxDataPoints=Ns_afe
  To Workspace5 : ToWorkspace  VariableName=ig_a_rms__mod1_sim  SampleTime=-1
      settings: MaxDataPoints=Ns_afe
  To Workspace6 : ToWorkspace  VariableName=ig_c_rms__mod1_sim  SampleTime=-1
      settings: MaxDataPoints=Ns_afe
  To Workspace7 : ToWorkspace  VariableName=pwr_act_grid_mod1_sim  SampleTime=-1
      settings: MaxDataPoints=Ns_afe
  To Workspace8 : ToWorkspace  VariableName=pwr_react_grid_mod1_sim  SampleTime=-1
      settings: MaxDataPoints=Ns_afe
  abc2alphabeta : Subsystem
  "abc2alphabeta " : Subsystem
  moving_avarage_p : Subsystem
  moving_avarage_q : Subsystem
  rms : Subsystem
  rms1 : Subsystem
  rms2 : Subsystem
  rms3 : Subsystem
  rms4 : Subsystem
  rms5 : Subsystem
  tag scope: cos_phi_avg=global, pwr_act_grid_mod1=global, pwr_react_grid_mod1=global
  wires:
  abc2alphabeta/2("beta ") -> Product1/1, Product2/1
  "abc2alphabeta "/2("beta ") -> Product1/2, Product3/1
  abc2alphabeta/1("alpha ") -> Product3/2, Product/1
  "abc2alphabeta "/1("alpha ") -> Product2/2, Product/2
  Product/1 -> Sum/1
  Product1/1 -> Sum/2
  Product2/1 -> Sum1/1
  Product3/1 -> Sum1/2
  Sum1/1 -> Gain3/1
  Sum/1 -> Gain2/1
  Gain2/1 -> moving_avarage_p/1(in), To Workspace7/1
  Gain3/1 -> To Workspace8/1, moving_avarage_q/1(in)
  [pwr_react_grid_mod1] -> Mux1/2
  Mux1/1 -> Fcn1/1
  Fcn1/1 -> [cos_phi_avg]
  [pwr_act_grid_mod1] -> Mux1/1
  rms/1(Out1) -> To Workspace2/1
  rms2/1(Out1) -> To Workspace3/1
  rms1/1(Out1) -> To Workspace1/1
  rms5/1(Out1) -> To Workspace6/1
  rms4/1(Out1) -> To Workspace4/1
  rms3/1(Out1) -> To Workspace5/1
  moving_avarage_p/1(out) -> Gain8/1
  moving_avarage_q/1(out) -> Gain9/1
  Demux2/1 -> Gain/1
  Demux2/2 -> Gain1/1
  Demux2/3 -> Gain4/1
  Demux3/1 -> Gain5/1
  Demux3/2 -> Gain6/1
  Demux3/3 -> Gain7/1
  Gain/1 -> rms/1(In1), abc2alphabeta/1(a)
  Gain1/1 -> rms1/1(In1), abc2alphabeta/2(b)
  Gain4/1 -> rms2/1(In1), abc2alphabeta/3(c)
  Gain5/1 -> rms3/1(In1), "abc2alphabeta "/1(a)
  Gain6/1 -> rms4/1(In1), "abc2alphabeta "/2(b)
  Gain7/1 -> rms5/1(In1), "abc2alphabeta "/3(c)
  Gain8/1 -> [pwr_act_grid_mod1]
  Gain9/1 -> [pwr_react_grid_mod1]
  [ugd_abc_pu_mod1] -> Demux2/1
  [igd_abc_pu_mod1] -> Demux3/1

== system afe_abc_inv_psm/afe_abc_inv_psm_mod1/AFE_control/afe_control/interesting scopes ==
  current_sequences_mod1 : Scope  NumInputPorts=4
      settings: ActiveDisplayYMinimum=-0.70787003636360168  ActiveDisplayYMaximum=0.41930654644966125  DataLoggingVariableName=ScopeData2
  i_grid_seq_ref : Scope
      settings: ActiveDisplayYMinimum=-1.125  ActiveDisplayYMaximum=0.125
  voltage_sequences_mod1 : Scope  NumInputPorts=4
      settings: ActiveDisplayYMinimum=-0.12510563433170316  ActiveDisplayYMaximum=1.1259507089853287
  wires:
  [v_grid_neg_eta_avg_mod1] -> voltage_sequences_mod1/4  "u_grid_neg_eta"
  [i_grid_neg_xi_avg_mod1] -> current_sequences_mod1/3  "i_grid_neg_xi"
  [v_grid_pos_eta_avg_mod1] -> voltage_sequences_mod1/2  "u_grid_pos_eta"
  [v_grid_neg_xi_avg_mod1] -> voltage_sequences_mod1/3  "u_grid_neg_xi"
  [i_grid_pos_xi_avg_mod1] -> current_sequences_mod1/1  "i_grid_pos_xi"
  [i_grid_neg_eta_avg_mod1] -> current_sequences_mod1/4  "i_grid_neg_eta"
  [v_grid_pos_xi_avg_mod1] -> voltage_sequences_mod1/1  "u_grid_pos_xi"
  [i_grid_pos_eta_avg_mod1] -> current_sequences_mod1/2  "i_grid_pos_eta"
  [i_grid_seq_ref_mod1] -> i_grid_seq_ref/1  "i_grid_seq_ref"

== system afe_abc_inv_psm/afe_abc_inv_psm_mod1/AFE_control/afe_control/is afe quantizzation and one step delay ==
  is_abc_pu : Inport
  Demux : Demux  Outputs=3
  Mux : Mux  Inputs=3
  is afe quantizzation and one step delay : Subsystem
  isd_abc_pu : Outport
  wires:
  is afe quantizzation and one step delay/2(isd_v_pu) -> Mux/2
  is_abc_pu/1 -> Demux/1
  is afe quantizzation and one step delay/3(isd_w_pu) -> Mux/3
  is afe quantizzation and one step delay/1(isd_u_pu) -> Mux/1
  Demux/1 -> is afe quantizzation and one step delay/1(is_u_pu)
  Mux/1 -> isd_abc_pu/1
  Demux/3 -> is afe quantizzation and one step delay/3(is_w_pu)
  Demux/2 -> is afe quantizzation and one step delay/2(is_v_pu)

== system afe_abc_inv_psm/afe_abc_inv_psm_mod1/AFE_control/afe_control/islanding_mode_detector ==
  gamma : Inport
  alpha : Inport  Port=2
  beta : Inport  Port=3
  Gain : Gain  Gain=7
  MATLAB Function : MATLAB Function  TreatAsAtomicUnit=on
  To Workspace20 : ToWorkspace  VariableName=u_7th_eta_sim_mod1  SampleTime=-1
      settings: MaxDataPoints=Ns_afe
  To Workspace21 : ToWorkspace  VariableName=u_7th_xi_sim_mod1  SampleTime=-1
      settings: MaxDataPoints=Ns_afe
  bounder : MATLAB Function  TreatAsAtomicUnit=on
  moving_avarage_1 : Subsystem
  moving_avarage_2 : Subsystem
  seventh_ugrid_component : Scope  NumInputPorts=2
      settings: ActiveDisplayYMinimum=-0.0034745064787606167  ActiveDisplayYMaximum=0.0074022094547510631  DataLoggingVariableName=ScopeData10
  tag scope: u_7th_eta_avg_mod1=global, u_7th_xi_avg_mod1=global
  wires:
  gamma/1 -> Gain/1  "gamma_grid"
  MATLAB Function/1(xi) -> moving_avarage_1/1(u)
  bounder/1(y) -> MATLAB Function/3(gamma)
  Gain/1 -> bounder/1(u)
  alpha/1 -> MATLAB Function/1(alpha)  "u_grid_alpha"
  beta/1 -> MATLAB Function/2(beta)  "u_grid_beta"
  MATLAB Function/2(eta) -> moving_avarage_2/1(u)
  [u_7th_xi_avg_mod1] -> To Workspace21/1
  [u_7th_eta_avg_mod1] -> To Workspace20/1
  moving_avarage_1/1(y) -> [u_7th_xi_avg_mod1], seventh_ugrid_component/1  "u_7th_xi"
  moving_avarage_2/1(y) -> [u_7th_eta_avg_mod1], seventh_ugrid_component/2  "u_7th_eta"

== system afe_abc_inv_psm/afe_abc_inv_psm_mod1/AFE_control/afe_control/phase_compensation_1 ==
  local_time : Inport
  master_time : Inport  Port=2
  alignment_eval_afe1 : Subsystem
  y : Outport
  wires:
  local_time/1 -> alignment_eval_afe1/1(local_time)
  master_time/1 -> alignment_eval_afe1/2(master_time)
  alignment_eval_afe1/1(dp) -> y/1

== system afe_abc_inv_psm/afe_abc_inv_psm_mod1/AFE_control/afe_control/space_vector ==
  uab_out : Inport
  Bus Creator : BusCreator  Inputs=3
  Bus Selector : BusSelector  OutputSignals=da,db,dc
  Bus Selector1 : BusSelector  OutputSignals=ualpha_afe,ubeta_afe
  C Caller : CCaller  FunctionName=sv_pwm_process_simulink  PortSpecificationStruct="%)30     .    V @   8    (     @         %    \"     4    !     0         %  0 \"0    $    _    07)G3F%M90  4&]R=$YA;64 4V-O<&4     26YD97@     5'EP90      4VEZ90      27-';&]B86P   X    P    !@    @    $          4    (     0    ,    !         !   P!O=70 #@   #     &    \"     0         !0    @    !     P    $         $  # &]U=  .    .     8    (    !          %    \"     $    &     0         0   ...(+2669 chars)"
  Constant : Constant  Value=ts_afe
  Constant1 : Constant
  Data Type Conversion1 : DataTypeConversion  OutDataTypeStr=double  SaturateOnIntegerOverflow=off  RndMeth=Floor
  Data Type Conversion15 : DataTypeConversion  OutDataTypeStr=single  SaturateOnIntegerOverflow=off  RndMeth=Floor
  Data Type Conversion16 : DataTypeConversion  OutDataTypeStr=single  SaturateOnIntegerOverflow=off  RndMeth=Floor
  Data Type Conversion17 : DataTypeConversion  OutDataTypeStr=uint32  SaturateOnIntegerOverflow=off  RndMeth=Floor
  Data Type Conversion18 : DataTypeConversion  OutDataTypeStr=single  SaturateOnIntegerOverflow=off  RndMeth=Floor
  Data Type Conversion2 : DataTypeConversion  OutDataTypeStr=double  SaturateOnIntegerOverflow=off  RndMeth=Floor
  Data Type Conversion3 : DataTypeConversion  OutDataTypeStr=double  SaturateOnIntegerOverflow=off  RndMeth=Floor
  Gain1 : Gain  Gain=sqrt(3)/2
  Gain2 : Gain  Gain=sqrt(3)/2
  duvw : Outport
  wires:
  Data Type Conversion15/1 -> C Caller/2
  Bus Selector/2 -> Data Type Conversion2/1  "<db>"
  Data Type Conversion16/1 -> C Caller/3
  Data Type Conversion18/1 -> C Caller/1
  C Caller/1 -> Bus Selector/1
  Bus Creator/1 -> duvw/1
  Data Type Conversion17/1 -> C Caller/4
  Data Type Conversion1/1 -> Bus Creator/1  "du(k)"
  Bus Selector1/2 -> Gain2/1  "<ubeta_afe>"
  Bus Selector/3 -> Data Type Conversion3/1  "<dc>"
  Bus Selector1/1 -> Gain1/1  "<ualpha_afe>"
  Data Type Conversion2/1 -> Bus Creator/2  "dv(k)"
  Gain2/1 -> Data Type Conversion15/1
  Bus Selector/1 -> Data Type Conversion1/1  "<da>"
  Gain1/1 -> Data Type Conversion18/1
  Data Type Conversion3/1 -> Bus Creator/3  "dw(k)"
  Constant/1 -> Data Type Conversion16/1
  uab_out/1 -> Bus Selector1/1
  Constant1/1 -> Data Type Conversion17/1

== system afe_abc_inv_psm/afe_abc_inv_psm_mod1/AFE_control/afe_control/udc_acquisition ==
  udc_pu : Inport
  Quantizer : Quantizer  QuantizationInterval=adc_quantization
  Unit Delay : UnitDelay  SampleTime=-1  HasFrameUpgradeWarning=on
  udcd_pu : Outport
  wires:
  Quantizer/1 -> Unit Delay/1
  udc_pu/1 -> Quantizer/1
  Unit Delay/1 -> udcd_pu/1

== system afe_abc_inv_psm/afe_abc_inv_psm_mod1/AFE_control/afe_control/udc_ctrl ==
  udc_pu : Inport
  udc_pu_ref : Inport  Port=2
  1/Ti : Gain  Gain=kp_vs  SaturateOnIntegerOverflow=on  OutDataTypeStr=Inherit: Same as input  ParamDataTypeStr=Inherit: Same as input
  Constant : Constant  Value=0
  Gain : Gain  Gain=-1
  Saturation : Saturate  UpperLimit=ixi_pos_ref_lim  LowerLimit=-ixi_pos_ref_lim
  Sum1 : Sum  Inputs=+++  SaturateOnIntegerOverflow=on
  Sum2 : Sum  Inputs=-+  SaturateOnIntegerOverflow=on
  Sum3 : Sum  Inputs=-+  SaturateOnIntegerOverflow=on
  Switch : Switch  Criteria=u2 > Threshold  SaturateOnIntegerOverflow=off  InputSameDT=off
  To Workspace1 : ToWorkspace  VariableName=udc_pu_sim_mod1  SampleTime=-1
      settings: MaxDataPoints=Ns_afe
  To Workspace3 : ToWorkspace  VariableName=udc_pu_ref_sim_mod1  SampleTime=-1
      settings: MaxDataPoints=Ns_afe
  Unit Delay4 : UnitDelay  SampleTime=-1  HasFrameUpgradeWarning=on
  kp : Gain  Gain=ki_vs*ts_afe  SaturateOnIntegerOverflow=on  OutDataTypeStr=Inherit: Same as input  ParamDataTypeStr=Inherit: Same as input
  udc_tracking : Scope  NumInputPorts=2
      settings: ActiveDisplayYMinimum=-0.14752197265624997  ActiveDisplayYMaximum=1.32769775390625  DataLoggingVariableName=ScopeData8
  i_xi_ref : Outport
  wires:
  1/Ti/1 -> Sum1/1, Sum3/1
  kp/1 -> Sum1/2
  Sum3/1 -> Unit Delay4/1
  Unit Delay4/1 -> Sum1/3
  udc_pu_ref/1 -> To Workspace3/1, udc_tracking/1, Sum2/2  "udc_pu_ref"
  udc_pu/1 -> To Workspace1/1, udc_tracking/2, Sum2/1  "udc_pu"
  Sum2/1 -> kp/1, 1/Ti/1
  Sum1/1 -> Saturation/1
  Saturation/1 -> Gain/1, Sum3/2
  [pwr_lim_enable_mod1] -> Switch/2
  Gain/1 -> Switch/3
  Switch/1 -> i_xi_ref/1
  Constant/1 -> Switch/1

== system afe_abc_inv_psm/afe_abc_inv_psm_mod1/AFE_control/afe_control/ug afe quantizzation and one step delay ==
  ug_abc_pu : Inport
  Demux : Demux  Outputs=3
  Mux : Mux  Inputs=3
  ug afe quantizzation and one step delay : Subsystem
  ugd_abc_pu : Outport
  wires:
  ug afe quantizzation and one step delay/2(ugd_v_pu) -> Mux/2
  Demux/2 -> ug afe quantizzation and one step delay/2(ug_v_pu)
  Demux/3 -> ug afe quantizzation and one step delay/3(ug_w_pu)
  ug afe quantizzation and one step delay/1(ugd_u_pu) -> Mux/1
  Demux/1 -> ug afe quantizzation and one step delay/1(ug_u_pu)
  ug_abc_pu/1 -> Demux/1
  ug afe quantizzation and one step delay/3(ugd_w_pu) -> Mux/3
  Mux/1 -> ugd_abc_pu/1

== system afe_abc_inv_psm/afe_abc_inv_psm_mod1/INV_control/inverter_control/Speed control ==
  rotor speed : Inport
  rotor speed ref : Inport  Port=2
  1/Ti : Gain  Gain=kp_w  SaturateOnIntegerOverflow=on  OutDataTypeStr=Inherit: Same as input  ParamDataTypeStr=Inherit: Same as input
  Saturation : Saturate  UpperLimit=iq_lim  LowerLimit=-iq_lim
  Sum1 : Sum  Inputs=+++  SaturateOnIntegerOverflow=on
  Sum2 : Sum  Inputs=-+  SaturateOnIntegerOverflow=on
  Sum3 : Sum  Inputs=-+  SaturateOnIntegerOverflow=on
  Unit Delay4 : UnitDelay  SampleTime=-1  HasFrameUpgradeWarning=on
  kp : Gain  Gain=ki_w*ts_inv  SaturateOnIntegerOverflow=on  OutDataTypeStr=Inherit: Same as input  ParamDataTypeStr=Inherit: Same as input
  torque_ref : Outport
  wires:
  1/Ti/1 -> Sum1/1, Sum3/1
  kp/1 -> Sum1/2
  Sum3/1 -> Unit Delay4/1
  Unit Delay4/1 -> Sum1/3
  rotor speed ref/1 -> Sum2/2
  rotor speed/1 -> Sum2/1
  Sum2/1 -> kp/1, 1/Ti/1
  Sum1/1 -> Saturation/1
  Saturation/1 -> Sum3/2, torque_ref/1

== system afe_abc_inv_psm/afe_abc_inv_psm_mod1/INV_control/inverter_control/current_ctrl ==
  torque_ref : Inport
  Bus Creator1 : BusCreator  Inputs=2
  bemf_observer : Subsystem
  current_ctrl : Subsystem
  current_transformation : Subsystem
  uab : Outport  VectorParamsAs1DForOutWhenUnconnected=off
  wires:
  [ubeta_pu_mod1] -> Bus Creator1/2  "ub"
  [ualpha_pu_mod1] -> Bus Creator1/1  "ua"
  Bus Creator1/1 -> uab/1
  torque_ref/1 -> current_ctrl/1(iq_ref)  "torque_ref"
  [ibeta_pu_mod1] -> bemf_observer/2(ibeta_pu)
  [ialpha_pu_mod1] -> bemf_observer/1(ialpha_pu)
  [ualpha_pu_mod1] -> bemf_observer/3(ualpha_pu)
  [ubeta_pu_mod1] -> bemf_observer/4(ubeta_pu)
  [udcd_pu_inv_mod1] -> current_ctrl/2(udc_pu), bemf_observer/5(udc_pu)
